simulink model "RC_transceiver_test"  (Simulink 7.5)
settings: Solver=FixedStepDiscrete  SolverMode=SingleTasking  StartTime=0.0  StopTime=10.0  FixedStep=0.01  RelTol=1e-3
undefined symbols (not defined in the file): DiscIntNeverNeededParam
libraries: dsPICdrivers x7, simulink x2
settings Model: Creator=Bryant  LastModifiedBy=Bryant
settings OptimizationCC: OptimizeModelRefInitCode=on  LifeSpan=1
settings HardwareCC: ProdBitPerInt=16  ProdEndianess=LittleEndian  ProdWordSize=16  ProdHWDeviceType=16-bit Generic
settings RTWCC: SystemTargetFile=dspic.tlc  MakeCommand=make_CreateMPLAB  TemplateMakefile=dspic_pic30_gcc.tmf  PostCodeGenCommand=dsPIC_Compile()  Description=Embedded Target for Microchip dsPIC (real-time)  ProcessScript=dspic_make_rtw_hook
settings CodeAppCC: IgnoreCustomStorageClasses=off
settings STFCustomTargetCC: IncludeMdlTerminateFcn=off  CombineOutputUpdateFcns=on  SuppressErrorStatus=on  ERTCustomFileBanners=on  SupportContinuousTime=off  SupportNonInlinedSFcns=off  SystemTargetFile=dspic.tlc
settings ERTTargetCC: MultiwordLength=2048  ParMdlRefBuildCompliant=off  CompOptLevelCompliant=off  IncludeMdlTerminateFcn=off  SuppressErrorStatus=on  ERTFirstTimeCompliant=off  ModelStepFunctionPrototypeControlCompliant=off  CPPClassGenCompliant=off  InlinedParameterPlacement=NonHierarchical  ERTSrcFileBannerTemplate=dsPIC_code_template.cgt  ERTHdrFileBannerTemplate=dsPIC_code_template.cgt  ERTDataSrcFileTemplate=dsPIC_code_template.cgt  ERTDataHdrFileTemplate=dsPIC_code_template.cgt  ERTCustomFileTemplate=dsPIC_main.tlc  ConvertIfToSwitch=off
settings CustomProperty: DataType=string  Value=C:\PROGRA~1\MATLAB\R2010a\bin\win64\gmake

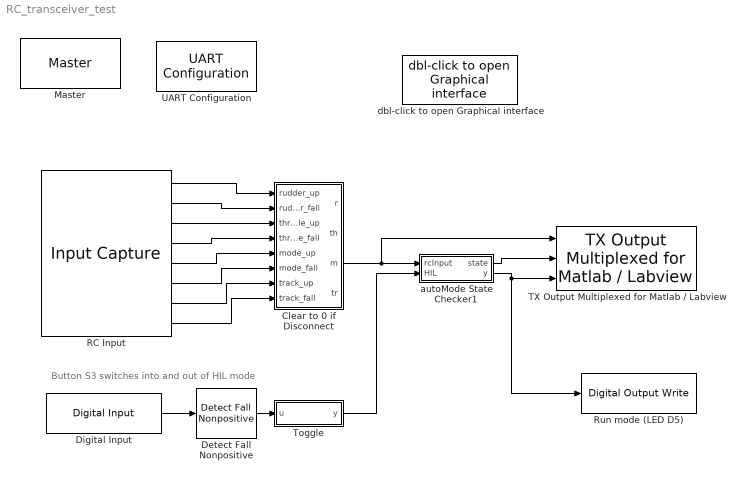
== system RC_transceiver_test ==
  note: Button S3 switches into and out of HIL mode
  Clear to 0 if Disconnect : Subsystem
  Detect Fall Nonpositive : simulink/Logic and Bit Operations/Detect Fall Nonpositive  SystemSampleTime=-1  vinit=1
  Digital Input : dsPICdrivers/Digital I//O/Digital Input  Tag=dsPIC_Digital_Input  PORT=D  Pin=[6]  SampleTime=.01  OrderingInOutPopup=None
  Master : dsPICdrivers/Master  Tag=dsPIC_MASTER  Priority=1  TimeStepType=Timer1  picType=33fJ256GP710  fcy=40000000  Quartz_33f=8e6  PLLActive_33f=on  fcyDesired_33f=40000000  tmr1="[8  49999  0]"  tmr1Info="Time Step : 0.01  ;   Error : 0%  PR1=49999"  tmr2345="[8  0  0  0  0  0  0  0]"  tmr2345cfg=[-1 -1 -1 -1 -1 -1 -1 -1]  IOautoConf=on  typePort="[ 0   0  10   0   0   0   0   0   0   0   0   0   0   0   0   0   0   0   0   0   0   0   0   0   0   0   0   0   0   0   0   0   0   0   0   0   0   0   0   0   0   0   0   0   0   0   0   0   0   0   0   0   0   0   9   0   0   6   6   6   0   0   0   6   0   0   0   0   0   0   0   0   0   0   0   0   0   0   0   0   0   0   0   0   4   5   0   0   0   0   0   0   0   0   0   0   0   0   0   0   0   0   0   0   0   0   0   0   0   0   0   0 ]"  TRIS="[ 65531  65535  65535  65535  65535  65535  65535 ]"  ADPCFG=0  MasterBusyPort=None  MasterOverloadPort=None  FOSC=Quartz (XT - HS)  ClockSwitchMonitor=Both disabled  TempProtection_33f=TEMP_ON  FPBOR=<empty>  PWRT=disable  MCLR=<empty>  ICD=ICS_PGD1  JTAGEN=JTAGEN_OFF  PowerSave=off  OverrideFcy=off  NewFcy=1e6  PR2345="[65535  65535  65535  65535  65535  65535  65535  65535]"
  RC Input : dsPICdrivers/Peripheral I//O/Input Capture  Tag=dsPIC_PWM_IC  IntPriority=7  Channel=[2 3 4 8]  Channel_UP_Down_Periode="[1  1  1  1]"  MaxChannel="[0.0025      0.0025      0.0025      0.0025]"  SafeMarge="[1  1  1  1]"  MaxName=' IC2max , IC3max , IC4max , IC8max '  Precision="[13.6094      13.6094      13.6094      13.6094]"  Timer="[2  2  2  2]"  ChangeDetected="[2  2  2  2]"  ChangeDetectedPortRef=3  SampleTime=.01  Status=OK
  Run mode (LED D5) : dsPICdrivers/Digital I//O/Digital Output Write  Tag=dsPIC_Digital_Output  Priority=5  PORT=A  Pin=[2]  Simultaneous=off  OrderingInOutPopup=None
  TX Output Multiplexed for Matlab / Labview : dsPICdrivers/Serial PORT/TX Output Multiplexed for Matlab // Labview  Tag=dsPIC_TX_Multiplexed  Priority=5  UART=2  CleverSpreadingChk=on  CleverSpreading=1  CHANNEL=[0 1 2]  CHANNELBLOCKED=[]  CHANNELBLOCKED_BITEWISE=0  Status=OK
  Toggle : Stateflow chart  TreatAsAtomicUnit=on
  UART Configuration : dsPICdrivers/Serial PORT/UART Configuration  Tag=dsPIC_config_UART  Priority=2  UART=2  proposed_BAUD=115200  BAUD=115200  ALT_TX_RX=off  InterruptTxWhen=When Transmit Buffer is empty  TXInterruptPri=1  TxBufferSize=32  TXEN=on  InterruptRxWhen=When Receive Buffer is full (contain 4 characters)  RXInterruptPri=2  RxBufferSize=32  DoNotImplementRxInterrupt=off  DoNotImplementTxInterrupt=off  UxBRG=21  Info="UxBRG = 21   ||  Real Baud : 113636   ||  % error : -1.3573  ||  max 113.6364 Bytes / Step"  RealBaud=0  ERROR=-1.3573  BYTES_STEP=113.6364
  autoMode State Checker1 : Stateflow chart  TreatAsAtomicUnit=on
  dbl-click to open Graphical interface : dsPICdrivers/Serial PORT/dbl-click to open Graphical interface  Nothing=0
  wires:
  Clear to 0 if Disconnect/3(m) -> autoMode State Checker1/1(rcInput), TX Output Multiplexed for Matlab / Labview/1
  RC Input/1 -> Clear to 0 if Disconnect/1(rudder_up)
  RC Input/2 -> Clear to 0 if Disconnect/2(rudder_fall)
  RC Input/3 -> Clear to 0 if Disconnect/3(throttle_up)
  RC Input/4 -> Clear to 0 if Disconnect/4(throttle_fall)
  RC Input/5 -> Clear to 0 if Disconnect/5(mode_up)
  RC Input/6 -> Clear to 0 if Disconnect/6(mode_fall)
  RC Input/7 -> Clear to 0 if Disconnect/7(track_up)
  RC Input/8 -> Clear to 0 if Disconnect/8(track_fall)
  Digital Input/1 -> Detect Fall Nonpositive/1
  Detect Fall Nonpositive/1 -> Toggle/1(u)
  autoMode State Checker1/2(y) -> TX Output Multiplexed for Matlab / Labview/3, Run mode (LED D5)/1
  autoMode State Checker1/1(state) -> TX Output Multiplexed for Matlab / Labview/2
  Toggle/1(y) -> autoMode State Checker1/2(HIL)

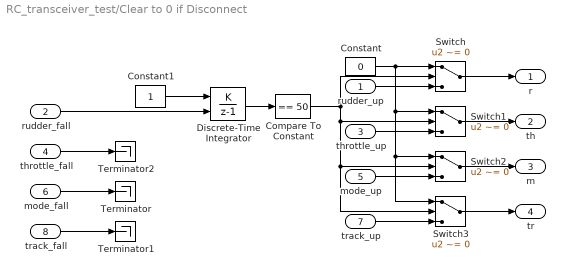
== system RC_transceiver_test/Clear to 0 if Disconnect ==
  rudder_up : Inport  OutDataType=sfix(16)  OutScaling=2^0
  rudder_fall : Inport  Port=2  OutDataType=sfix(16)  OutScaling=2^0
  throttle_up : Inport  Port=3  OutDataType=sfix(16)  OutScaling=2^0
  throttle_fall : Inport  Port=4  OutDataType=sfix(16)  OutScaling=2^0
  mode_up : Inport  Port=5  OutDataType=sfix(16)  OutScaling=2^0
  mode_fall : Inport  Port=6  OutDataType=sfix(16)  OutScaling=2^0
  track_up : Inport  Port=7  OutDataType=sfix(16)  OutScaling=2^0
  track_fall : Inport  Port=8  OutDataType=sfix(16)  OutScaling=2^0
  Compare To Constant : simulink/Logic and Bit Operations/Compare To Constant  SystemSampleTime=-1  relop===  const=50  LogicOutDataTypeMode=boolean
  Constant : Constant  Value=0  OutDataTypeMode=uint16  OutDataType=sfix(16)  OutScaling=2^0  OutDataTypeStr=uint16
  Constant1 : Constant  OutDataTypeMode=uint8  OutDataType=fixdt(1, 16)  OutScaling=2^0  OutDataTypeStr=uint8
  Discrete-Time Integrator : DiscreteIntegrator  IntegratorMethod=Accumulation: Forward Euler  ExternalReset=level  SampleTime=-1  OutDataType=fixdt(1, 16)  OutScaling=2^0  LimitOutput=on  UpperSaturationLimit=50  LowerSaturationLimit=0  ICPrevOutput=DiscIntNeverNeededParam  ICPrevScaledInput=DiscIntNeverNeededParam
  Switch{,1..3} (4 alike) : Switch  Criteria=u2 ~= 0  Threshold=40
  Terminator : Terminator
  Terminator1 : Terminator
  Terminator2 : Terminator
  r : Outport  OutDataType=sfix(16)  OutScaling=2^0
  th : Outport  Port=2  OutDataType=sfix(16)  OutScaling=2^0
  m : Outport  Port=3  OutDataType=sfix(16)  OutScaling=2^0
  tr : Outport  Port=4  OutDataType=sfix(16)  OutScaling=2^0
  wires:
  Switch1/1 -> th/1
  throttle_up/1 -> Switch1/3
  Switch/1 -> r/1
  rudder_up/1 -> Switch/3
  Constant/1 -> Switch/1, Switch1/1, Switch2/1, Switch3/1
  Switch2/1 -> m/1
  mode_up/1 -> Switch2/3
  track_up/1 -> Switch3/3
  Switch3/1 -> tr/1
  Compare To Constant/1 -> Switch/2, Switch1/2, Switch2/2, Switch3/2
  rudder_fall/1 -> Discrete-Time Integrator/2
  mode_fall/1 -> Terminator/1
  track_fall/1 -> Terminator1/1
  Constant1/1 -> Discrete-Time Integrator/1
  throttle_fall/1 -> Terminator2/1
  Discrete-Time Integrator/1 -> Compare To Constant/1

== matlab function autoMode State Checker1 ==
  data: state output double; rcInput input double; y output double; HIL input double
function [state,y]  = fcn(rcInput, HIL)
%#eml

% Initialize a persistent state variable that initializes to -1, the startup
% state value.
persistent internalState;
if isempty(internalState)
    internalState = int8(-1);
end

% Implement the state machine.
switch internalState
    case -1 % Startup
        if rcInput ~= 0
            if rcInput > 7000
                internalState = int8(0);
            else
                internalState = int8(1);
            end
        elseif HIL
            internalState = int8(1);
        end
    case 0 % Manual mode
        if rcInput ~= 0
            if rcInput > 7000
                internalState = int8(0);
            else
                internalState = int8(1);
            end
        elseif HIL
            internalState = int8(1);
        end
    case 1 % Autonomous mode
        if rcInput ~= 0
            if rcInput > 7000
                internalState = int8(0);
            else
                internalState = int8(1);
            end
        end
end

% Here the current autonomous state is output as either 1:"on" or 0:"off"
if internalState == int8(1)
    y = true;
else
    y = false;
end
state = internalState;

== matlab function Toggle ==
  data: u input double; y output double
function y = toggle(u)
%#eml

persistent pre_output;

% Initialize pre_output
if isempty(pre_output)
    pre_output = false;
end

% If we receive the toggle input, toggle
if u
    if pre_output
        pre_output = false;
    else
        pre_output = true;
    end
end

y = pre_output;
